simulink model "microgrid_with_PPWFFN"  (R2024b)
settings: Solver=VariableStepAuto  StartTime=0.0  StopTime=5  RelTol=1e-3
libraries: eeTransforms x2, spsDCVoltageSourceLib x1, eePwmGeneratorTwoLevel x1, eePowerMeasurement x1, eeSinusoidalMeasurement x1, spsThreePhaseParallelRLCBranchLib x1, spsThreePhaseParallelRLCLoadLib x1, spsThreePhaseSeriesRLCBranchLib x1, spsThreePhaseVIMeasurementLib x1, spsThreePhaseBreakerLib x1, spsUniversalBridgeLib x1, slpidlib x1
settings Model: Creator=visnn  LastModifiedBy=visnn

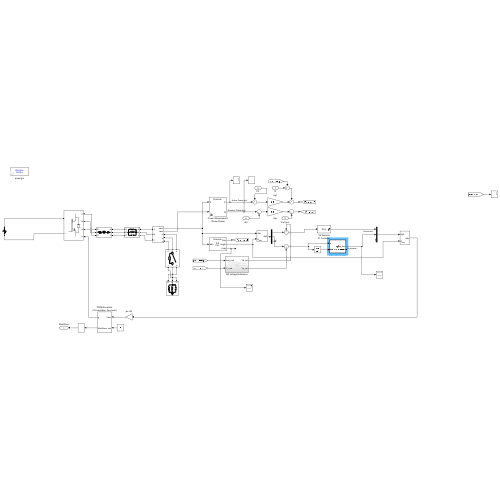
[thumbnail: Simulink's stored preview of the top-level diagram]
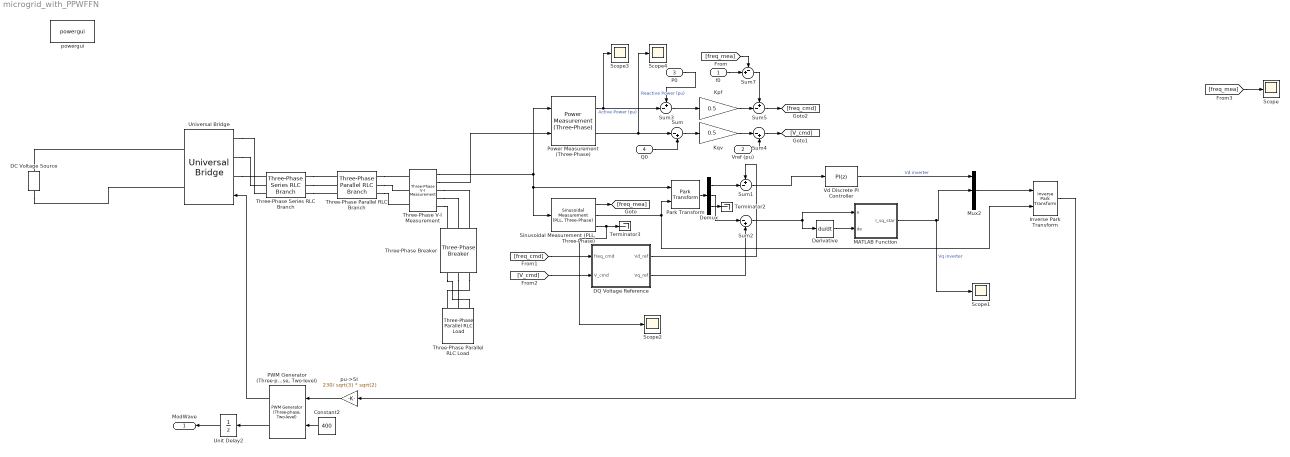
== system microgrid_with_PPWFFN ==
  f0 : Inport
  Vref (pu) : Inport  Port=2
  P0 : Inport  Port=3
  Q0 : Inport  Port=4
  Constant2 : Constant  Value=400
  DC Voltage Source : spsDCVoltageSourceLib/DC Voltage Source  Amplitude=400  Measurements=None
  DQ Voltage Reference : Subsystem
  Demux : Demux  Outputs=3
  Derivative : Derivative
  Inverse Park Transform : eeTransforms/Inverse Park Transform  AxisAlignment=Q-axis  PowerInvariant=off
  Kpf : Gain  Gain=0.5
  Kqv : Gain  Gain=0.5
  MATLAB Function : MATLAB Function  TreatAsAtomicUnit=on
  Mux2 : Mux  Inputs=3
  "PWM Generator (Three-phase, Two-level)" : eePwmGeneratorTwoLevel/PWM Generator (Three-phase, Two-level)  PWMMode=Continuous PWM (CPWM)  CPWMMode=SPWM: sinusoidal PWM  DPWMMode=60 DPWM: 60 degree discontinuous PWM  fsw=10000  Ts=1e-5
  Park Transform : eeTransforms/Park Transform  AxisAlignment=Q-axis  PowerInvariant=off
  Power Measurement (Three-Phase) : eePowerMeasurement/Power Measurement (Three-Phase)  LabelModeActiveChoice=Discrete  F=50  K=1  Seq=Positive  Ts=1e-4
  Scope{,1..4} (5 alike) : Scope
  "Sinusoidal Measurement (PLL, Three-Phase)" : eeSinusoidalMeasurement/Sinusoidal Measurement (PLL, Three-Phase)  Kp_LF=180  Ki_LF=3200  F0=50  Theta0=0  Ts=1e-5
  Sum : Sum  Inputs=|-+
  Sum1 : Sum  Inputs=+-|  InputSameDT=on  SaturateOnIntegerOverflow=on  OutDataTypeStr=Inherit: Same as first input
  Sum2 : Sum  Inputs=|-+  InputSameDT=on  SaturateOnIntegerOverflow=on  OutDataTypeStr=Inherit: Same as first input
  Sum3 : Sum  Inputs=+-|
  Sum4 : Sum  Inputs=|-+
  Sum5 : Sum  Inputs=+-|
  Sum7 : Sum  Inputs=-+|
  Terminator2 : Terminator
  Terminator3 : Terminator
  Three-Phase Parallel RLC Branch : spsThreePhaseParallelRLCBranchLib/Three-Phase Parallel RLC Branch  LConnTagsString=A|B|C  RConnTagsString=A|B|C  BranchType=RLC  Resistance=1  Inductance=1e-3  Capacitance=1e-6  Measurements=None
  Three-Phase Parallel RLC Load : spsThreePhaseParallelRLCLoadLib/Three-Phase Parallel RLC Load  LConnTagsString=A|B|C  Configuration=Y (grounded)  NominalVoltage=1000  Vabc=[1e3 1e3 1e3]  Vabcp=[1e3 1e3 1e3]  NominalFrequency=60  UnbalancedPower=off  ActivePower=10e3  InductivePower=100  CapacitivePower=100  Pabc=[10e3 9e3 11e3]  QLabc=[100 90 110]  QCabc=[100 90 110]  Pabcp=[10e3 9e3 11e3]  QLabcp=[100 90 110]  QCabcp=[100 90 110]  Measurements=None  LoadType=constant Z
  Three-Phase Series RLC Branch : spsThreePhaseSeriesRLCBranchLib/Three-Phase Series RLC Branch  LConnTagsString=A|B|C  RConnTagsString=A|B|C  BranchType=RLC  Resistance=1  Inductance=0.005  Capacitance=1e-6  Measurements=None
  Three-Phase V-I Measurement : spsThreePhaseVIMeasurementLib/Three-Phase V-I Measurement  VoltageMeasurement=phase-to-ground  SetLabelV=off  LabelV=Vabc  Vpu=off  VpuLL=off  CurrentMeasurement=yes  SetLabelI=off  LabelI=Iabc  Ipu=off  Pbase=100e6  Vbase=500e3  OutputType=Complex  PhasorSimulation=off  PSBequivalent=0
  Three-Phase Breaker : spsThreePhaseBreakerLib/Three-Phase Breaker  InitialState=open  SwitchA=on  SwitchB=on  SwitchC=on  SwitchTimes="[1/60  5/60]"  External=off  BreakerResistance=0.01  SnubberResistance=1e6  SnubberCapacitance=inf  Measurements=None
  Unit Delay2 : UnitDelay  SampleTime=1e-5  HasFrameUpgradeWarning=on
  Universal Bridge : spsUniversalBridgeLib/Universal Bridge  Arms=3  SnubberResistance=1e5  SnubberCapacitance=inf  Device=IGBT / Diodes  Ron=1e-3  Lon=0  ForwardVoltages="[  0  0  ]"  ForwardVoltage=0  GTOparameters=[ 10e-6 , 20e-6 ]  IGBTparameters=[ 1e-6 , 2e-6 ]  Measurements=None  Measurements_2=None  converterType=Rectifier
  Vd Discrete PI Controller : slpidlib/PID Controller  Controller=PI  Form=Parallel  TimeDomain=Discrete-time  UseExternalTs=off  SampleTime=1e-5  IntegratorMethod=Forward Euler  FilterMethod=Forward Euler  ControllerParametersSource=internal  P=1.0  I=0.01  UseKiTs=off  D=0  UseExternalDerivativeSource=off  N=100  UseFilter=on  TunerSelectOption=Transfer Function Based (PID Tuner App)  InitialConditionSource=internal  InitialConditionForIntegrator=0  InitialConditionForFilter=0  DifferentiatorICPrevScaledInput=0  ExternalReset=none  TrackingMode=off  Kt=1  LimitOutput=on  SatLimitsSource=internal  UpperSaturationLimit=1  LowerSaturationLimit=0  LinearizeAsGain=on  AntiWindupMode=none  Kb=1  LimitIntegrator=off  UpperIntegratorSaturationLimit=inf  LowerIntegratorSaturationLimit=-inf  POutMin=[]  POutMax=[]  IOutMin=[]  IOutMax=[]  DOutMin=[]  DOutMax=[]  NOutMin=[]  NOutMax=[]  SumOutMin=[]  SumOutMax=[]  SaturationOutMin=[]  SaturationOutMax=[]  PParamMin=[]  PParamMax=[]  IParamMin=[]  IParamMax=[]  DParamMin=[]  DParamMax=[]  NParamMin=[]  NParamMax=[]  KbParamMin=[]  KbParamMax=[]  KtParamMin=[]  KtParamMax=[]  KbOutMin=[]  KbOutMax=[]  KtOutMin=[]  KtOutMax=[]  IntegratorOutMin=[]  IntegratorOutMax=[]  FilterOutMin=[]  FilterOutMax=[]  SumI1OutMin=[]  SumI1OutMax=[]  SumI2OutMin=[]  SumI2OutMax=[]  SumI3OutMin=[]  SumI3OutMax=[]  SumI4OutMin=[]  SumI4OutMax=[]  SumDOutMin=[]  SumDOutMax=[]  DifferentiatorOutMin=[]  DifferentiatorOutMax=[]  FilterDiffOutCoefMin=[]  FilterDiffOutCoefMax=[]  ReciprocalOutMin=[]  ReciprocalOutMax=[]  SumDenOutMin=[]  SumDenOutMax=[]  SumNumOutMin=[]  SumNumOutMax=[]  DivideOutMin=[]  DivideOutMax=[]  UdiffTsProdOutMin=[]  UdiffTsProdOutMax=[]  NTsProdOutMin=[]  NTsProdOutMax=[]  UintegralTsProdOutMin=[]  UintegralTsProdOutMax=[]  UngainTsProdOutMin=[]  UngainTsProdOutMax=[]  ClampingZeroOutDataTypeStr=Inherit: Inherit via back propagation  ClampingZeroOutMin=[]  ClampingZeroOutMax=[]  FilterDenConstantOutDataTypeStr=Inherit: Inherit via back propagation  FilterDenConstantOutMin=[]  FilterDenConstantOutMax=[]  PCopyOutDataTypeStr=Inherit: Inherit via back propagation  PCopyOutMin=[]  PCopyOutMax=[]  NCopyOutDataTypeStr=Inherit: Inherit via back propagation  NCopyOutMin=[]  NCopyOutMax=[]  IntegratorContinuousStateAttributes=''  IntegratorStateMustResolveToSignalObject=off  IntegratorRTWStateStorageClass=Auto  FilterContinuousStateAttributes=''  FilterStateMustResolveToSignalObject=off  FilterRTWStateStorageClass=Auto  ParallelPVariant=InternalParameters  IdealPVariant=Disabled  IVariant=InternalParameters  DVariant=Disabled  IntegratorVariant=Discrete  SatVariant=Enabled  AWVariant=Passthrough  PCopyVariant=Disabled  TRVariant=Disabled  FdbkBlocksVariant=Forward  IdealPFdbkVariant=Disabled  SatFdbkVariant=Disabled  DerivativeFilterVariant=Disabled  NVariant=Disabled  NCopyVariant=Disabled_SignalSpec  FilterICVariant=Disabled  IntegratorICVariant=InternalICs  ExternalResetVariant=Disabled  TRSumVariant=Passthrough  SumFdbkVariant=Disabled  SumVariant=Sum_PI  TsampFilterVariant=InternalTs  TsampNgainVariant=Passthrough  TsampIntegralVariant=Disabled_SignalSpec  ExternalSaturationOutDataTypeStr=Inherit: Same as second input  DerivativeSourceVariant=Disabled  PreIntVariant=InternalPreInt
  powergui : sps_lib/powergui  Priority=1  SimulationMode=Discrete  SampleTime=1e-5  frequency=60  Iterations=50  frequencyindice=0  Pbase=100e6  ErrMax=1e-4  UnitsV=kV  UnitsW=MW  buscounter=0  FunctionMessages=off  echomessages=off  EnableUseOfTLC=off  CurrentSourceSwitches=off  DisableSnubberDevices=off  DisableRonSwitches=off  DisableVfSwitches=off  DisplayEquations=off  AutomaticDiscreteSolvers=off  SolverType=Tustin/Backward Euler (TBE)  Interpol=off  ExternalGateDelay=off  methode=off  Ts=100  x0status=blocks  SPID=on  SwTol=0  HookPort=off  NonlinearTolerance=1e-4  nMaxIteration=100  ContinueOnMaxIteration=off  RestoreLinks=warning  ResistiveCurrentMeasurement=off  Frange=[0:2:500]  Ylog=off  Xlog=on  ShowGrid=off  save=off  variable=ZData  structure=0  ZoomFFT=off  StartTime=0.0  cycles=1  DisplayStyle=1  fundamental=60  FreqAxis=off  MaxFrequency=1000  frequencyindicesteady=1  RmsSteady=1  display=off
  pu->SI : Gain  Gain=230/ sqrt(3) * sqrt(2)
  ModWave : Outport
  wires:
  "Sinusoidal Measurement (PLL, Three-Phase)"/2 -> Park Transform/2, Inverse Park Transform/2
  "PWM Generator (Three-phase, Two-level)"/1 -> Universal Bridge/1
  "Sinusoidal Measurement (PLL, Three-Phase)"/1 -> [freq_mea]
  Power Measurement (Three-Phase)/2 -> Sum/1, Scope4/1  "Reactive Power (pu)"
  Three-Phase V-I Measurement/1 -> Park Transform/1, "Sinusoidal Measurement (PLL, Three-Phase)"/1, Power Measurement (Three-Phase)/1
  Mux2/1 -> Inverse Park Transform/1
  Sum5/1 -> [freq_cmd]
  Q0/1 -> Sum/2
  Sum/1 -> Kqv/1
  Vd Discrete PI Controller/1 -> Mux2/1  "Vd inverter"
  pu->SI/1 -> "PWM Generator (Three-phase, Two-level)"/1
  DQ Voltage Reference/2(Vq_ref) -> Sum2/2
  P0/1 -> Sum3/1
  Constant2/1 -> "PWM Generator (Three-phase, Two-level)"/2
  Unit Delay2/1 -> ModWave/1
  Park Transform/1 -> Demux/1
  Vref (pu)/1 -> Sum4/2
  Demux/2 -> Sum2/1
  Sum3/1 -> Kpf/1
  f0/1 -> Sum7/2
  "PWM Generator (Three-phase, Two-level)"/2 -> Unit Delay2/1
  Demux/3 -> Terminator2/1
  Inverse Park Transform/1 -> pu->SI/1
  [freq_cmd] -> DQ Voltage Reference/1(freq_cmd)
  Three-Phase V-I Measurement/2 -> Power Measurement (Three-Phase)/2
  DQ Voltage Reference/1(Vd_ref) -> Sum1/1
  Power Measurement (Three-Phase)/1 -> Scope3/1, Sum3/2  "Active Power (pu)"
  Sum7/1 -> Sum5/1
  [freq_mea] -> Sum7/1
  Kpf/1 -> Sum5/2
  [V_cmd] -> DQ Voltage Reference/2(V_cmd)
  Demux/1 -> Sum1/2
  "Sinusoidal Measurement (PLL, Three-Phase)"/3 -> Scope2/1, Terminator3/1
  Kqv/1 -> Sum4/1
  Sum4/1 -> [V_cmd]
  Sum1/1 -> Vd Discrete PI Controller/1
  Sum2/1 -> Derivative/1, MATLAB Function/1(e)
  MATLAB Function/1(I_sq_star) -> Scope1/1, Mux2/2  "Vq inverter"
  [freq_mea] -> Scope/1
  Derivative/1 -> MATLAB Function/2(de)
  connections:
  Three-Phase Breaker/RConn1 -- Three-Phase Parallel RLC Load/LConn1
  Three-Phase Parallel RLC Branch/RConn2 -- Three-Phase V-I Measurement/LConn2
  Universal Bridge/LConn1 -- Three-Phase Series RLC Branch/LConn1
  Three-Phase V-I Measurement/RConn1 -- Three-Phase Breaker/LConn1
  Universal Bridge/LConn3 -- Three-Phase Series RLC Branch/LConn3
  DC Voltage Source/RConn1 -- Universal Bridge/RConn1
  Three-Phase Breaker/RConn3 -- Three-Phase Parallel RLC Load/LConn3
  Three-Phase Series RLC Branch/RConn2 -- Three-Phase Parallel RLC Branch/LConn2
  Three-Phase Series RLC Branch/RConn3 -- Three-Phase Parallel RLC Branch/LConn3
  Three-Phase Parallel RLC Branch/RConn3 -- Three-Phase V-I Measurement/LConn3
  Three-Phase V-I Measurement/RConn2 -- Three-Phase Breaker/LConn2
  Universal Bridge/LConn2 -- Three-Phase Series RLC Branch/LConn2
  Three-Phase Series RLC Branch/RConn1 -- Three-Phase Parallel RLC Branch/LConn1
  Three-Phase Breaker/RConn2 -- Three-Phase Parallel RLC Load/LConn2
  DC Voltage Source/LConn1 -- Universal Bridge/RConn2
  Three-Phase Parallel RLC Branch/RConn1 -- Three-Phase V-I Measurement/LConn1
  Three-Phase V-I Measurement/RConn3 -- Three-Phase Breaker/LConn3

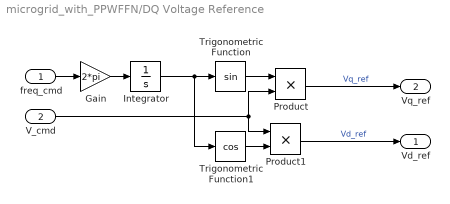
== system microgrid_with_PPWFFN/DQ Voltage Reference ==
  freq_cmd : Inport
  V_cmd : Inport  Port=2
  Gain : Gain  Gain=2*pi
  Integrator : Integrator
  Product : Product
  Product1 : Product
  Trigonometric Function : Trigonometry
  Trigonometric Function1 : Trigonometry  Operator=cos
  Vd_ref : Outport
  Vq_ref : Outport  Port=2
  wires:
  Product/1 -> Vq_ref/1  "Vq_ref"
  Product1/1 -> Vd_ref/1  "Vd_ref"
  Trigonometric Function/1 -> Product/1
  V_cmd/1 -> Product/2, Product1/1
  Integrator/1 -> Trigonometric Function/1, Trigonometric Function1/1
  freq_cmd/1 -> Gain/1
  Trigonometric Function1/1 -> Product1/2
  Gain/1 -> Integrator/1

== matlab function microgrid_with_PPWFFN/MATLAB Function ==
  settings: updateMethod=DISCRETE
  data: e input; I_sq_star output; de input
function I_sq_star = PPWFNN_Controller(e, de)

% === Layer 1: Input Layer ===
x1 = [e; de];   % Inputs: e and de

% === Layer 2: Membership Layer (Gaussian functions) ===
% Parameters (6 neurons): means and std deviations (initialized)
m2 = [-0.6, -0.3, 0, 0.3, 0.6, 0.9];
sigma2 = 0.2 * ones(1, 6);

% Gaussian fuzzification for both e and de (2 x 6)
y2_e = exp(-((x1(1) - m2).^2) ./ (sigma2.^2));
y2_de = exp(-((x1(2) - m2).^2) ./ (sigma2.^2));

% Combine both dimensions into single activation (6 rules max for now)
y2 = y2_e .* y2_de;  % Simple product rule for 2D MF

% === Layer 3: Petri Layer ===
% Dynamic threshold
F = 0.5 * (x1(1) + x1(2));
alpha = 1; beta = 2;
dth = (alpha * exp(-beta * F)) / (1 + exp(-beta * F));
t3 = double(y2 >= dth);  % Transition firing

y3 = y2 .* t3;

% === Layer 4: Probabilistic Layer ===
% Simulated Gaussian kernel again (with fixed mean/variance)
m4 = linspace(-1, 1, 6);  % Simplified
sigma4 = 0.3;
y4 = exp(-((y3 - m4).^2) / sigma4^2);

% === Layer 5: Wavelet Layer ===
% Mexican hat wavelet
m5 = m4; sigma5 = 0.4;
phi = 1 ./ sqrt(abs(sigma5)) .* ...
    (1 - ((x1(1) - m5).^2) ./ sigma5.^2) .* ...
    exp(-((x1(1) - m5).^2) ./ (2 * sigma5.^2));

% === Layer 6: Rule Layer ===
% Combine all layers into final rule output
rule_out = y2 .* y3 .* y4 .* phi;

% === Layer 7: Output Layer ===
% Weighted sum of rule outputs (weights w7)
w7 = [1.2, 0.9, -0.5, 0, 0.7, 1.1];  % Tunable weights
I_sq_star = sum(w7 .* rule_out);

end
